simulink model "quadrotor_1"  (R2021a)
settings: Solver=VariableStepAuto  StartTime=0.0  StopTime=20  RelTol=1e-3
undefined symbols (not defined in the file): dpitch, droll, dx, dy, dyaw, dz, normrnd, pitch, pitch_sen, quadrotor, roll, roll_sen, rot2, X, X_sen, Y, Y_sen, yaw, yaw_sen, Z, Z_sen
libraries: simulink x1
settings Model: Creator=Evgeniy  LastModifiedBy=Evgeniy

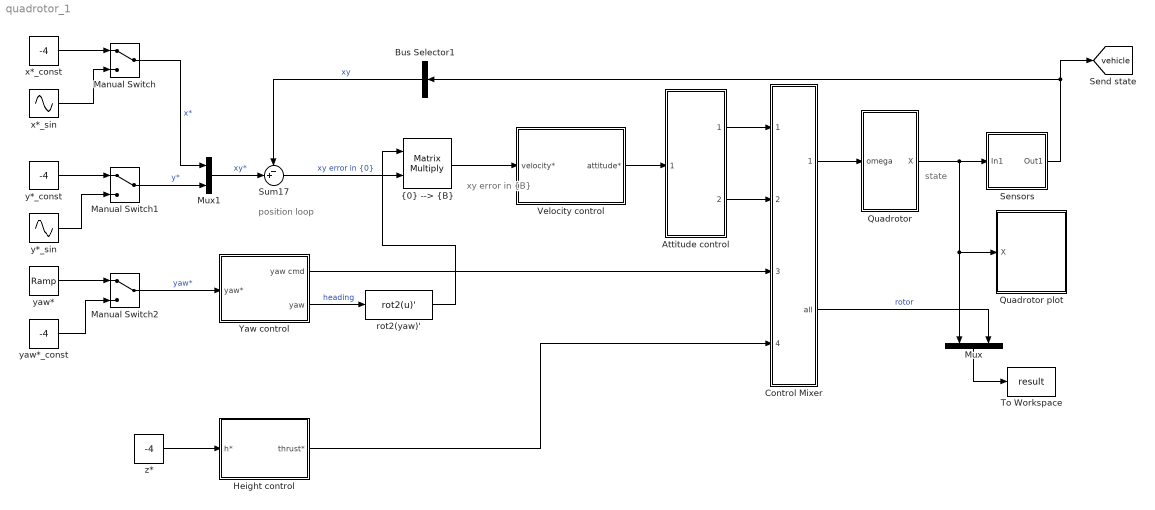
== system quadrotor_1 ==
  note: state
  note: xy error
      | in {B}
  note: position
      | loop
  Attitude control : Subsystem  mask{P=100, D=1}
      mask prompts: P "Proportional gain"; D "Derivative gain"
  Bus Selector1 : BusSelector  OutputSignals=X_sen,Y_sen  OutputAsBus=on
  Control Mixer : Subsystem  mask{quad=quadrotor, maxrot=1000, minrot=5}
      mask prompts: quad "Quadrotor parameters"; maxrot "Maximum rotor speed (rad/s)"; minrot "Minimum rotor speed (rad/s)"
      mask help: Quadrotor control mixer
      mask Help:
      | Determine rotor speeds based on desired torques and thrust, and propellor model
      | 
      | <b>Inputs::</b>
      | tau<sub>x</sub> (1x1)    desired rolling torque [Nm]
      | 
      | tau<sub>y</sub> (1x1)    desired pitching torque [Nm]
      | tau<sub>z</sub> (1x1)    desired yawing torque [Nm]
      | T (1x1)          desired thrust [N]
      | 
      | <b>Outputs::</b>
      | 
      | w1 (1x1) angular velocity of rotor 1 [rad]
      | w2 (1x1) angular velocity of rotor 2 [rad]
      | w3 (1x1) angular velocity of rotor 3 [rad]
      | w4 (1x1) angular velocity of rotor 4 [rad]
      | 
      | <b>Notes::</b>
      | 
      | - Assumes the rotor labelling convention of RVC Fig 4.16.
      | - The quadrotor is underactuated and has only 4 inputs.
      mask Display:
      | port_label('output',1,'\varpi','texmode','on');
      | port_label('output',2,'\tau_a','texmode','on');
      | port_label('input',1,'\tau_x','texmode','on');
      | port_label('input',2,'\tau_y','texmode','on');
      | port_label('input',3,'\tau_z','texmode','on');
      | port_label('input',4,'T','texmode','on');
  Height control : Subsystem  mask{P=4, D=1, T0=40}
      mask prompts: P "Proportional gain"; D "Derivative gain"; T0 "Thrust feedforward"
  Manual Switch : ManualSwitch
  Manual Switch1 : ManualSwitch
  Manual Switch2 : ManualSwitch
  Mux : Mux  Inputs=2
  Mux1 : Mux  Inputs=2
  Quadrotor : Subsystem  mask{quad=quadrotor, x0=[0 0 -0.2], groundflag=on}
      mask prompts: quad "Quadrotor params"; x0 "Initial position"; groundflag "Ground"
      mask help: Quadrotor dynamics
      mask Help:
      | Integrate spatial velocity to update pose represented as a homogeneous
      | transformation.
      | 
      | <b>Parameters::</b>
      | 
      | q (struct)  A structure containing quadrotor dynamics
      | 
      | The elements of q are:
      | 
      |  J         Flyer rotational inertia matrix (3x3)
      |  h         Height of rotors above CoG (1x1)
      |  d         Length of flyer arms (1x1)
      |  nb        Number of blades per rotor (1x1)
      |  r         Rotor radius (1x1)
      |  c         Blade chord (1x1)
      |  e         Flapping hinge offset (1x1)
      |  Mb        Rotor blade mass (1x1)
      |  Mc        Estimated hub clamp mass (1x1)
      |  ec        Blade root clamp displacement (1x1)
      |  Ib        Rotor blade rotational inertia (1x1)
      |  Ic        Estimated root clamp inertia (1x1)
      |  mb        Static blade moment (1x1)
      |  Ir        Total rotor inertia (1x1)
      |  Ct        Non-dim. thrust coefficient (1x1)
      |  Cq        Non-dim. torque coefficient (1x1)
      |  sigma     Rotor solidity ratio (1x1)
      |  thetat    Blade tip angle (1x1)
      |  theta0    Blade root angle (1x1)
      |  theta1    Blade twist angle (1x1)
      |  theta75   3/4 blade angle (1x1)
      |  thetai    Blade ideal root approximation (1x1)
      |  a         Lift slope gradient (1x1)
      |  A         Rotor disc area (1x1)
      |  gamma     Lock number (1x1)
      | 
      | 
      | <b>Inputs::</b>
      | 
      | w1 (1x1) angular velocity of rotor 1 [rad]
      | w2 (1x1) angular velocity of rotor 2 [rad]
      | w3 (1x1) angular velocity of rotor 3 [rad]
      | w4 (1x1) angular velocity of rotor 4 [rad]
      | 
      | <b>Outputs::</b>
      | 
      | X (1x12) state vector (x, y, z, thr, thp, thy, xd, yd, zd, thrd, thpd, thyd)
      | 
      | (x,y,z) is the position in the world frame [m]
      | (thr, thp, thy) the roll/pitch/yaw orientation in the world frame [rad]
      | (xd,yd,zd) is the velocity in the body frame [m]
      | (thrd,thpd,thyd) is the roll/pitch/yaw rates in the body frame [rad/s]
      | 
      | <b>Notes::</b>
      | 
      | - See also mdl_quadrotor which defines parameters for the ANU X4 flyer.
      mask Display:
      | port_label('input',1,'\varpi','texmode','on');
      | port_label('output',1,'X','texmode','on');
  Quadrotor plot : Subsystem  mask{quad=quadrotor, xydim=5, zdim=10}
      mask prompts: quad "Model"; xydim "xy-axes dimension"; zdim "z-axis dimension"
      mask help: Animate quadrotor.
      mask Help:
      | This block graphically displays a quadrotor (flying robot).
      | 
      | A new figure is created and A graphical model of a quadrotor is animated
      | to a pose specified by the state vector input to the block.
      | 
      | The state vector is [x y z roll pitch yaw] in world coordinates and the
      | angles are in radians.
      | 
      | Notes:
      | - The dimensions of the vehicle workspace are set by parameters
  Sensors : Subsystem  mask{x_sen_sigma=1, y_sen_sigma=1, z_sen_sigma=1, yaw_sen_sigma=1, pitch_sen_sigma=1, roll_sen_sigma=1}
      mask help:
      | Block for adding noise to signals.
      | Noise has a Gaussian distribution.
      mask Help: Help of Test sensor block
      mask Display:
      | port_label('input',1,'i','texmode','on');
      | port_label('output',1,'o','texmode','on');
  Sum17 : Sum  Inputs=-+|
  To Workspace : ToWorkspace  VariableName=result  SampleTime=-1
  Velocity control : Subsystem  mask{P=0.1, D=2}
      mask prompts: P "Proportional gain"; D "Derivative gain"
  Yaw control : Subsystem  mask{P=20, D=2}
      mask prompts: P "Proportional gain"; D "Derivative gain"
  rot2(yaw)' : MATLABFcn  MATLABFcn=rot2(u)'  OutputDimensions=[2 2]  Output1D=off
  x*_const : Constant  Value=-4  SampleTime=0
  x*_sin : Sin  Frequency=2*pi*.125  Phase=-pi/2  SampleTime=0
  y*_const : Constant  Value=-4  SampleTime=0
  y*_sin : Sin  Frequency=2*pi*.125  Phase=-pi/2  SampleTime=0
  yaw* : simulink/Sources/Ramp  slope=0.2  start=2  InitialOutput=0
  yaw*_const : Constant  Value=-4  SampleTime=0
  z* : Constant  Value=-4  SampleTime=0
  "{0} --> {B}" : Product  Multiplication=Matrix(*)  RndMeth=Zero
  tag scope: vehicle=global
  wires:
  Yaw control/1(yaw cmd) -> Control Mixer/3(tau yaw)
  Height control/1(thrust*) -> Control Mixer/4(total thrust)
  Mux1/1 -> Sum17/2  "xy*"
  Attitude control/1(roll torque*) -> Control Mixer/1(tau roll)
  Bus Selector1/1 -> Sum17/1  "xy"
  Control Mixer/1(omega) -> Quadrotor/1(omega)
  "{0} --> {B}"/1 -> Velocity control/1(velocity*)
  z*/1 -> Height control/1(h*)
  Mux/1 -> To Workspace/1
  Quadrotor/1(X) -> Quadrotor plot/1(X), Mux/1, Sensors/1(In1)
  rot2(yaw)'/1 -> "{0} --> {B}"/1
  Velocity control/1(attitude*) -> Attitude control/1(attitude*)
  Control Mixer/2(all) -> Mux/2  "rotor"
  Sum17/1 -> "{0} --> {B}"/2  "xy error in {0}"
  Yaw control/2(yaw) -> rot2(yaw)'/1  "heading"
  Attitude control/2(pitch torque*) -> Control Mixer/2(tau pitch)
  x*_const/1 -> Manual Switch/1
  x*_sin/1 -> Manual Switch/2
  Manual Switch/1 -> Mux1/1  "x*"
  y*_const/1 -> Manual Switch1/1
  y*_sin/1 -> Manual Switch1/2
  Manual Switch1/1 -> Mux1/2  "y*"
  Sensors/1(Out1) -> [vehicle], Bus Selector1/1
  yaw*/1 -> Manual Switch2/1
  Manual Switch2/1 -> Yaw control/1(yaw*)  "yaw*"
  yaw*_const/1 -> Manual Switch2/2

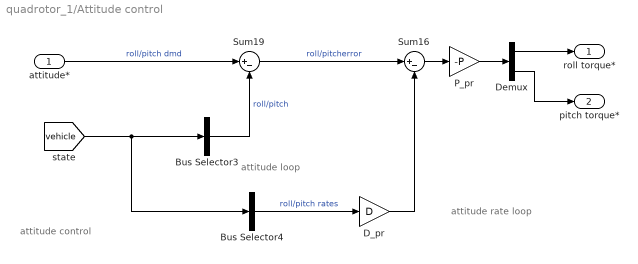
== system quadrotor_1/Attitude control ==
  note: attitude control
  note: attitude rate loop
  note: attitude loop
  attitude* : Inport
  Bus Selector3 : BusSelector  OutputSignals=roll,pitch  OutputAsBus=on
  Bus Selector4 : BusSelector  OutputSignals=droll,dpitch  OutputAsBus=on
  D_pr : Gain  Gain=D
  Demux : Demux  Outputs=2
  P_pr : Gain  Gain=-P
  Sum16 : Sum  Inputs=|+-
  Sum19 : Sum  Inputs=|+-
  roll torque* : Outport
  pitch torque* : Outport  Port=2
  wires:
  [vehicle] -> Bus Selector4/1, Bus Selector3/1
  attitude*/1 -> Sum19/1  "roll/pitch dmd"
  Bus Selector3/1 -> Sum19/2  "roll/pitch"
  Bus Selector4/1 -> D_pr/1  "roll/pitch rates"
  Sum19/1 -> Sum16/1  "roll/pitcherror"
  Sum16/1 -> P_pr/1
  P_pr/1 -> Demux/1
  D_pr/1 -> Sum16/2
  Demux/2 -> pitch torque*/1
  Demux/1 -> roll torque*/1

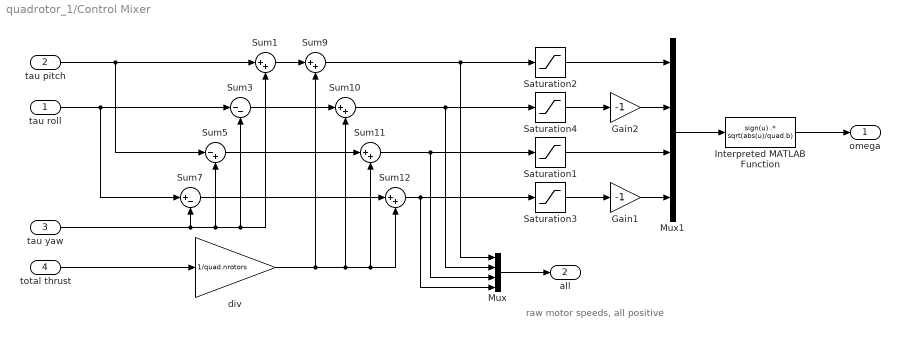
== system quadrotor_1/Control Mixer ==
  note: raw motor speeds, all positive
  tau roll : Inport
  tau pitch : Inport  Port=2
  tau yaw : Inport  Port=3
  total thrust : Inport  Port=4
  Gain1 : Gain  Gain=-1
  Gain2 : Gain  Gain=-1
  Interpreted MATLAB Function : MATLABFcn  MATLABFcn=sign(u) .* sqrt(abs(u)/quad.b)
  Mux : Mux
  Mux1 : Mux
  Saturation{1..4} (4 alike) : Saturate  UpperLimit=maxrot  LowerLimit=minrot  ZeroCross=off
  Sum{1,9..12} (5 alike) : Sum  Inputs=|++  InputSameDT=on  SaturateOnIntegerOverflow=on  OutDataTypeStr=Inherit: Same as first input
  Sum3 : Sum  Inputs=|--  InputSameDT=on  SaturateOnIntegerOverflow=on  OutDataTypeStr=Inherit: Same as first input
  Sum5 : Sum  Inputs=|-+  InputSameDT=on  SaturateOnIntegerOverflow=on  OutDataTypeStr=Inherit: Same as first input
  Sum7 : Sum  Inputs=|+-  InputSameDT=on  SaturateOnIntegerOverflow=on  OutDataTypeStr=Inherit: Same as first input
  div : Gain  Gain=1/quad.nrotors
  omega : Outport  VectorParamsAs1DForOutWhenUnconnected=off
  all : Outport  Port=2  VectorParamsAs1DForOutWhenUnconnected=off
  wires:
  div/1 -> Sum11/2, Sum12/2, Sum10/2, Sum9/2
  Interpreted MATLAB Function/1 -> omega/1
  Mux1/1 -> Interpreted MATLAB Function/1
  Gain2/1 -> Mux1/2
  tau yaw/1 -> Sum7/2, Sum5/2, Sum3/2, Sum1/2
  Saturation2/1 -> Mux1/1
  Saturation4/1 -> Gain2/1
  Saturation1/1 -> Mux1/3
  Saturation3/1 -> Gain1/1
  tau pitch/1 -> Sum1/1, Sum5/1
  Sum1/1 -> Sum9/1
  Sum3/1 -> Sum10/1
  Sum5/1 -> Sum11/1
  Sum7/1 -> Sum12/1
  Sum9/1 -> Saturation2/1, Mux/1
  Sum10/1 -> Mux/2, Saturation4/1
  Sum11/1 -> Mux/3, Saturation1/1
  Sum12/1 -> Mux/4, Saturation3/1
  total thrust/1 -> div/1
  tau roll/1 -> Sum3/1, Sum7/1
  Mux/1 -> all/1
  Gain1/1 -> Mux1/4

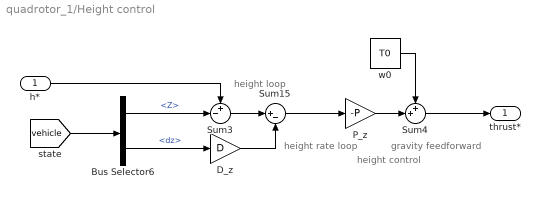
== system quadrotor_1/Height control ==
  note: height control
  note: gravity feedforward
  note: height rate
      | loop
  note: height
      | loop
  h* : Inport
  Bus Selector6 : BusSelector  OutputSignals=Z,dz
  D_z : Gain  Gain=D
  P_z : Gain  Gain=-P
  Sum15 : Sum  Inputs=|+-
  Sum3 : Sum  Inputs=+-|
  Sum4 : Sum  Inputs=++|
  w0 : Constant  Value=T0  SampleTime=0
  thrust* : Outport
  wires:
  w0/1 -> Sum4/1
  Sum15/1 -> P_z/1
  P_z/1 -> Sum4/2
  Bus Selector6/1 -> Sum3/2  "<Z>"
  h*/1 -> Sum3/1
  Sum3/1 -> Sum15/1
  Bus Selector6/2 -> D_z/1  "<dz>"
  D_z/1 -> Sum15/2
  Sum4/1 -> thrust*/1
  [vehicle] -> Bus Selector6/1

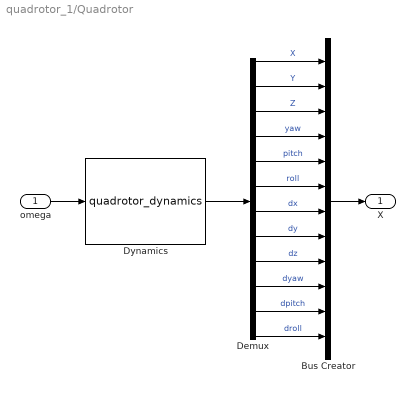
== system quadrotor_1/Quadrotor ==
  omega : Inport
  Bus Creator : BusCreator  Inputs='X','Y','Z','yaw','pitch','roll','dx','dy','dz','dyaw','dpitch','droll'
  Demux : Demux  Outputs=12
      settings: DisplayOption=none
  Dynamics : S-Function  FunctionName=quadrotor_dynamics  Parameters=quad, x0, groundflag  SFunctionDeploymentMode=off  EnableBusSupport=off
  X : Outport  VectorParamsAs1DForOutWhenUnconnected=off
  wires:
  Demux/1 -> Bus Creator/1  "X"
  Demux/3 -> Bus Creator/3  "Z"
  Demux/4 -> Bus Creator/4  "yaw"
  Demux/5 -> Bus Creator/5  "pitch"
  omega/1 -> Dynamics/1
  Demux/7 -> Bus Creator/7  "dx"
  Demux/9 -> Bus Creator/9  "dz"
  Demux/2 -> Bus Creator/2  "Y"
  Demux/6 -> Bus Creator/6  "roll"
  Demux/8 -> Bus Creator/8  "dy"
  Bus Creator/1 -> X/1
  Dynamics/1 -> Demux/1
  Demux/10 -> Bus Creator/10  "dyaw"
  Demux/11 -> Bus Creator/11  "dpitch"
  Demux/12 -> Bus Creator/12  "droll"

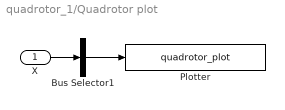
== system quadrotor_1/Quadrotor plot ==
  X : Inport
  Bus Selector1 : BusSelector  OutputSignals=X,Y,Z,yaw,pitch,roll  OutputAsBus=on
  Plotter : S-Function  FunctionName=quadrotor_plot  Parameters=[xydim, zdim], 1, 1,quad  SFunctionDeploymentMode=off  EnableBusSupport=off
  wires:
  X/1 -> Bus Selector1/1
  Bus Selector1/1 -> Plotter/1

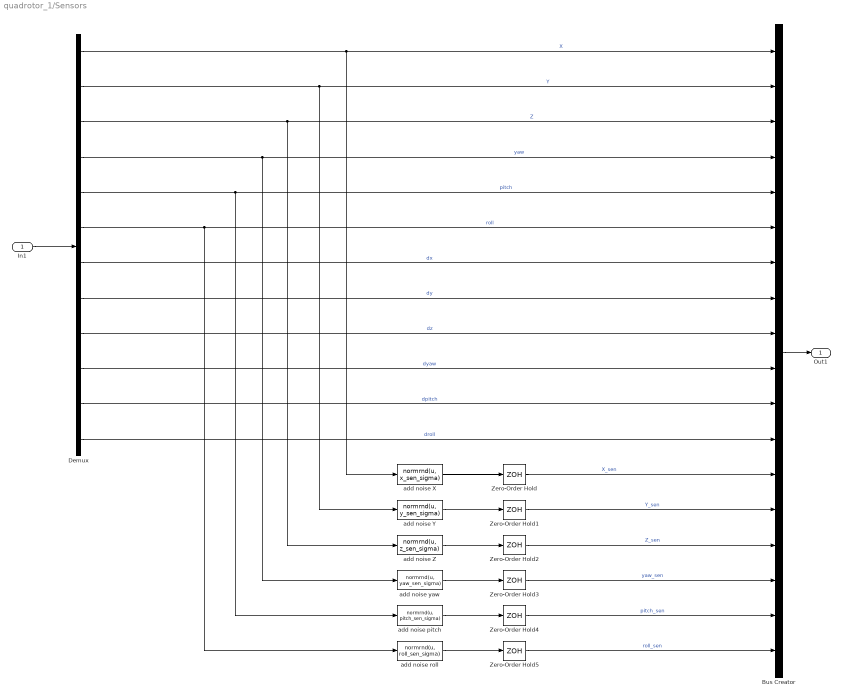
== system quadrotor_1/Sensors ==
  In1 : Inport
  Bus Creator : BusCreator  Inputs=X,Y,Z,yaw,pitch,roll,dx,dy,dz,dyaw,dpitch,droll,X_sen,Y_sen,Z_sen,yaw_sen,pitch_sen,roll_sen
  Demux : Demux  Outputs=12
      settings: DisplayOption=none
  Zero-Order Hold{,1..5} (6 alike) : ZeroOrderHold  SampleTime=0.01
  add noise X : MATLABFcn  MATLABFcn=normrnd(u, x_sen_sigma)
  add noise Y : MATLABFcn  MATLABFcn=normrnd(u, y_sen_sigma)
  add noise Z : MATLABFcn  MATLABFcn=normrnd(u, z_sen_sigma)
  add noise pitch : MATLABFcn  MATLABFcn=normrnd(u, pitch_sen_sigma)
  add noise roll : MATLABFcn  MATLABFcn=normrnd(u, roll_sen_sigma)
  add noise yaw : MATLABFcn  MATLABFcn=normrnd(u, yaw_sen_sigma)
  Out1 : Outport
  wires:
  Demux/5 -> add noise pitch/1, Bus Creator/5  "pitch"
  Bus Creator/1 -> Out1/1
  Demux/4 -> add noise yaw/1, Bus Creator/4  "yaw"
  Demux/7 -> Bus Creator/7  "dx"
  Demux/11 -> Bus Creator/11  "dpitch"
  Demux/3 -> add noise Z/1, Bus Creator/3  "Z"
  Demux/6 -> add noise roll/1, Bus Creator/6  "roll"
  Demux/1 -> add noise X/1, Bus Creator/1  "X"
  Demux/10 -> Bus Creator/10  "dyaw"
  Demux/2 -> add noise Y/1, Bus Creator/2  "Y"
  Demux/8 -> Bus Creator/8  "dy"
  Demux/12 -> Bus Creator/12  "droll"
  In1/1 -> Demux/1
  Demux/9 -> Bus Creator/9  "dz"
  add noise X/1 -> Zero-Order Hold/1
  add noise Y/1 -> Zero-Order Hold1/1
  add noise Z/1 -> Zero-Order Hold2/1
  add noise yaw/1 -> Zero-Order Hold3/1
  add noise pitch/1 -> Zero-Order Hold4/1
  add noise roll/1 -> Zero-Order Hold5/1
  Zero-Order Hold/1 -> Bus Creator/13  "X_sen"
  Zero-Order Hold1/1 -> Bus Creator/14  "Y_sen"
  Zero-Order Hold2/1 -> Bus Creator/15  "Z_sen"
  Zero-Order Hold3/1 -> Bus Creator/16  "yaw_sen"
  Zero-Order Hold4/1 -> Bus Creator/17  "pitch_sen"
  Zero-Order Hold5/1 -> Bus Creator/18  "roll_sen"

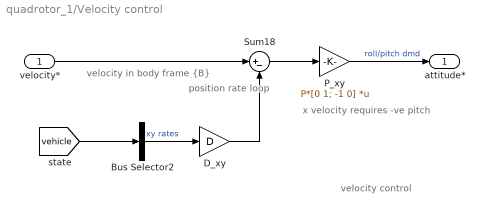
== system quadrotor_1/Velocity control ==
  note: x velocity requires -ve pitch
  note: velocity in body frame {B}
  note: velocity control
  note: position rate
      | loop
  velocity* : Inport
  Bus Selector2 : BusSelector  OutputSignals=dx,dy  OutputAsBus=on
  D_xy : Gain  Gain=D
  P_xy : Gain  Gain=P*[0 1; -1 0]  Multiplication=Matrix(K*u)
  Sum18 : Sum  Inputs=|+-
  attitude* : Outport
  wires:
  Bus Selector2/1 -> D_xy/1  "xy rates"
  D_xy/1 -> Sum18/2
  Sum18/1 -> P_xy/1
  velocity*/1 -> Sum18/1
  [vehicle] -> Bus Selector2/1
  P_xy/1 -> attitude*/1  "roll/pitch dmd"

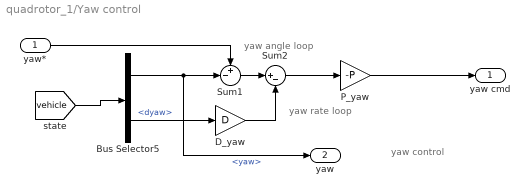
== system quadrotor_1/Yaw control ==
  note: yaw control
  note: yaw rate
      | loop
  note: yaw angle
      | loop
  yaw* : Inport
  Bus Selector5 : BusSelector  OutputSignals=yaw,dyaw
  D_yaw : Gain  Gain=D
  P_yaw : Gain  Gain=-P
  Sum1 : Sum  Inputs=+-|
  Sum2 : Sum  Inputs=|+-
  yaw cmd : Outport
  yaw : Outport  Port=2
  wires:
  [vehicle] -> Bus Selector5/1
  P_yaw/1 -> yaw cmd/1
  Bus Selector5/1 -> yaw/1, Sum1/2  "<yaw>"
  Sum2/1 -> P_yaw/1
  Bus Selector5/2 -> D_yaw/1  "<dyaw>"
  D_yaw/1 -> Sum2/2
  Sum1/1 -> Sum2/1
  yaw*/1 -> Sum1/1
